simulink model "Parcial1Punto2"  (R2017b)
settings: Solver=VariableStepAuto  StartTime=0.0  StopTime=10.0  RelTol=1e-3
settings Model: Creator=Cx001la  LastModifiedBy=Cx001la

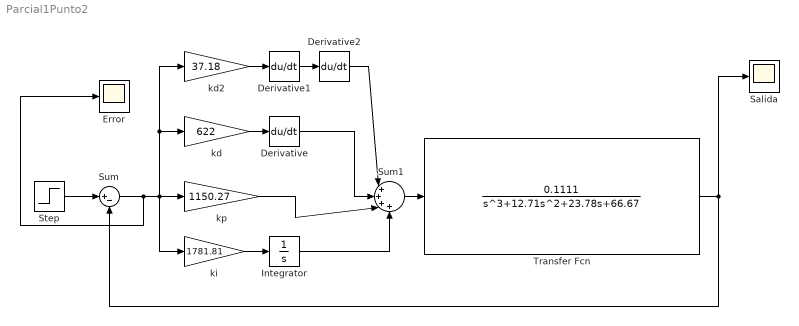
== system Parcial1Punto2 ==
  Derivative : Derivative
  Derivative1 : Derivative
  Derivative2 : Derivative
  Error : Scope
  Integrator : Integrator
  Salida : Scope
  Step : Step  Time=0  SampleTime=0
  Sum : Sum  Inputs=|+-
  Sum1 : Sum  Inputs=|++++
  Transfer Fcn : TransferFcn  Numerator=[0.1111]  Denominator=[1 12.71 23.78 66.67]
  kd : Gain  Gain=622
  kd2 : Gain  Gain=37.18
  ki : Gain  Gain=1781.81
  kp : Gain  Gain=1150.27
  wires:
  Derivative1/1 -> Derivative2/1
  kd2/1 -> Derivative1/1
  kd/1 -> Derivative/1
  Derivative2/1 -> Sum1/1
  Derivative/1 -> Sum1/2
  kp/1 -> Sum1/3
  Integrator/1 -> Sum1/4
  ki/1 -> Integrator/1
  Sum1/1 -> Transfer Fcn/1
  Sum/1 -> Error/1, ki/1, kd2/1, kd/1, kp/1
  Step/1 -> Sum/1
  Transfer Fcn/1 -> Salida/1, Sum/2
